simulink model "opc_simple_teste"  (R2013a)
settings: Solver=ode45  StartTime=0.0  StopTime=4500  RelTol=1e-3
undefined symbols (not defined in the file or in its folder): Bomba1, Bomba2, Opc_Teste, Tanq1, Tanq2, Tanq3, Tanq4
libraries: opclib x3
settings Model: Creator=Administrator  LastModifiedBy=Administrator

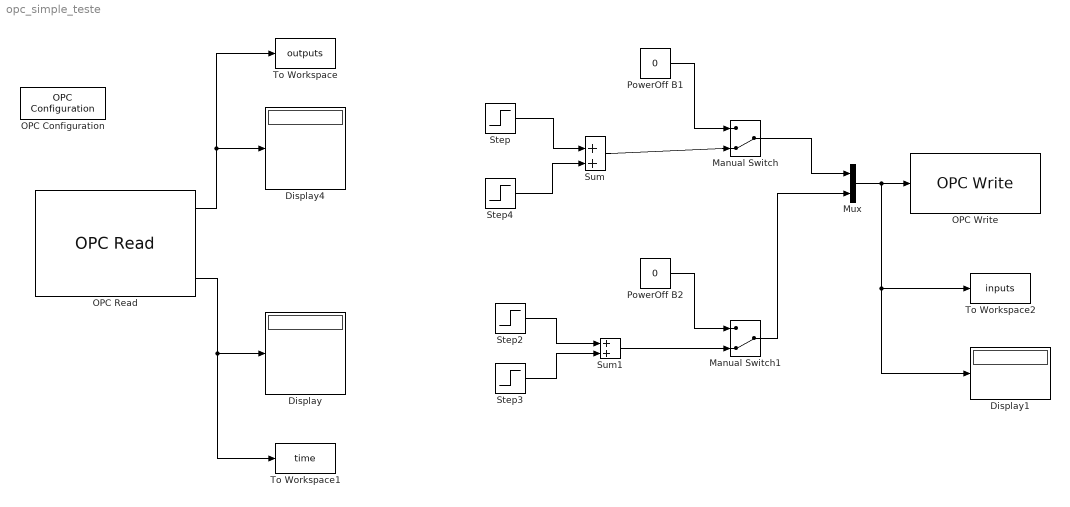
== system opc_simple_teste ==
  Display : Display
  Display1 : Display
  Display4 : Display
  Manual Switch : ManualSwitch  CurrentSetting=0
  Manual Switch1 : ManualSwitch  CurrentSetting=0
  Mux : Mux  Inputs=2
  OPC Configuration : opclib/OPC Configuration  opcServers=localhost/RSLinx OPC Server/10  errMissingItems=Error  errReadWrite=Warn  errShutdown=Error  errRTViolation=Warn  rtEnable=on  speedup=1  showLatency=off  beingUsed=on
  OPC Read : opclib/OPC Read  serverHost=localhost  serverID=RSLinx OPC Server  itemIDs=[Opc_Teste]Tanq4, [Opc_Teste]Tanq3, [Opc_Teste]Tanq2, [Opc_Teste]Tanq1  readMode=Synchronous (cache)  dataType=double  updateRate=0.2  showQual=on  showTS=on  tsMode=Seconds since start
  OPC Write : opclib/OPC Write  serverHost=localhost  serverID=RSLinx OPC Server  itemIDs=[Opc_Teste]Bomba1, [Opc_Teste]Bomba2  writeMode=Synchronous  updateRate=0.2
  PowerOff B1 : Constant  Value=0
  PowerOff B2 : Constant  Value=0
  Step : Step  Time=1500  Before=42  After=45
  Step2 : Step  Time=3000  Before=42  After=45
  Step3 : Step  Time=4000  After=-45
  Step4 : Step  Time=4000  After=-45
  Sum : Sum  Inputs=+|+
  Sum1 : Sum  Inputs=+|+
  To Workspace : ToWorkspace  VariableName=outputs  SampleTime=-1  SaveFormat=Timeseries
  To Workspace1 : ToWorkspace  VariableName=time  SampleTime=-1  SaveFormat=Timeseries
  To Workspace2 : ToWorkspace  VariableName=inputs  SampleTime=-1  SaveFormat=Timeseries
  wires:
  OPC Read/3 -> To Workspace1/1, Display/1
  OPC Read/1 -> To Workspace/1, Display4/1
  PowerOff B1/1 -> Manual Switch/1
  PowerOff B2/1 -> Manual Switch1/1
  Sum1/1 -> Manual Switch1/2
  Manual Switch/1 -> Mux/1
  Manual Switch1/1 -> Mux/2
  Mux/1 -> Display1/1, To Workspace2/1, OPC Write/1
  Sum/1 -> Manual Switch/2
  Step2/1 -> Sum1/1
  Step3/1 -> Sum1/2
  Step4/1 -> Sum/2
  Step/1 -> Sum/1
